simulink model "sampleModel1579_1_sub_sub"  (R2023a)
settings: Solver=VariableStepAuto  StartTime=0.0  StopTime=10.0  RelTol=1e-3
libraries: hdlsllib x7, simulink x2
settings Model: Creator=user1  LastModifiedBy=user1
settings OptimizationCC: BlockReduction=off  ConditionallyExecuteInputs=off

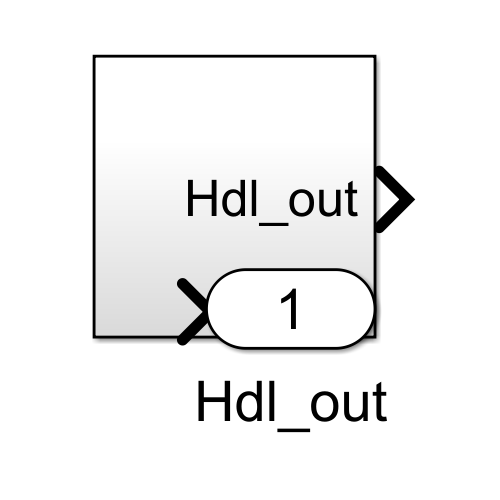
[thumbnail: Simulink's stored preview of the top-level diagram]
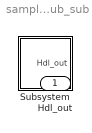
== system sampleModel1579_1_sub_sub ==
  Subsystem : Subsystem
  Hdl_out : Outport  OutDataTypeStr=uint8

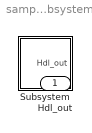
== system sampleModel1579_1_sub_sub/Subsystem ==
  Subsystem : Subsystem
  Hdl_out : Outport  OutDataTypeStr=uint8

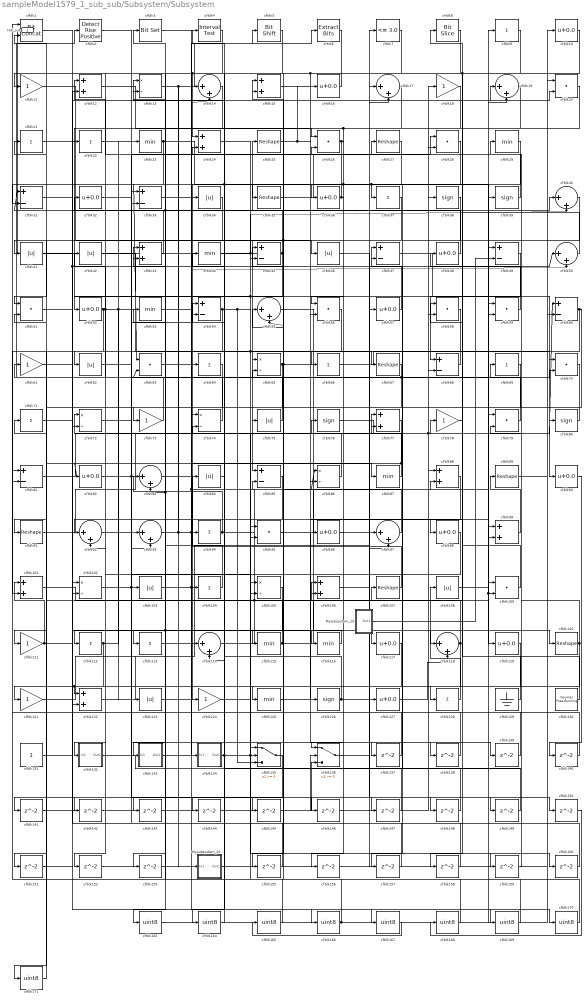
== system sampleModel1579_1_sub_sub/Subsystem/Subsystem ==
  Mysubsystem_13 : Subsystem  TreatAsAtomicUnit=on  RTWFcnName=Mysubsystem_13
      settings: RTWFcnNameOpts=User specified  RTWFileNameOpts=Use function name
  Mysubsystem_20 : Subsystem  TreatAsAtomicUnit=on  RTWFcnName=Mysubsystem_20
      settings: RTWFcnNameOpts=User specified  RTWFileNameOpts=Use function name
  cfblk1 : hdlsllib/Logic and Bit Operations/Bit Concat  numInputs=2
  cfblk{10,16,32,36,48,52,57,82,90,96,98,117,119,127} (14 alike) : Bias  Bias=0.0  SaturateOnIntegerOverflow=off
  cfblk{12,15,24,43,77,88,99,101,106,122} (10 alike) : Sum  OutDataTypeStr=uint8
  cfblk{13,65,72,74,86,102,105} (7 alike) : Product  Inputs=*/  OutDataTypeStr=uint8  RndMeth=Zero  SaturateOnIntegerOverflow=on
  cfblk{34,41..42,46,62,75,84,103,108,123} (10 alike) : Abs  OutDataTypeStr=uint8  SaturateOnIntegerOverflow=off
  cfblk{9,21..22,37,64,66,69,71,94,104,112..113,128} (13 alike) : Sum  Inputs=+  OutDataTypeStr=uint8
  cfblk{25,27,35,67,89,91,107,120} (8 alike) : Reshape
  cfblk{20,26,28,51,56,58..59,63,70,79,95,109} (12 alike) : DotProduct  OutDataTypeStr=uint8
  cfblk{11,18,61,73,78,111,121,124} (8 alike) : Gain  OutDataTypeStr=uint8
  cfblk{14,17,19,40,50,55,83,92..93,97,114,118} (12 alike) : Sum  Inputs=|++  OutDataTypeStr=uint8
  cfblk{23,29,44,53,87,115..116,125} (8 alike) : MinMax  OutDataTypeStr=uint8
  cfblk{38..39,76,80,126} (5 alike) : Signum
  cfblk129 : Ground
  cfblk130 : hdlsllib/Sources/Counter Free-Running  NumBits=16  tsamp=-1
  cfblk131 : Constant  OutDataTypeStr=uint8  SampleTime=-1
  cfblk132 : Subsystem
      settings: LibrarySourceBlock=|
      | hdlsllib/Ports &
      | Subsystems/Subsystem
  cfblk133 : Subsystem
      settings: LibrarySourceBlock=|
      | hdlsllib/Ports &
      | Subsystems/Subsystem
  cfblk134 : Subsystem
      settings: LibrarySourceBlock=|
      | hdlsllib/Ports &
      | Subsystems/Subsystem
  cfblk135 : Switch  OutDataTypeStr=uint8  SaturateOnIntegerOverflow=off  InputSameDT=off
  cfblk136 : Switch  OutDataTypeStr=uint8  SaturateOnIntegerOverflow=off  InputSameDT=off
  cfblk{137..153,155..160} (23 alike) : Delay  SampleTime=1
  cfblk{163..171} (9 alike) : DataTypeConversion  OutDataTypeStr=uint8  SaturateOnIntegerOverflow=off  RndMeth=Floor
  cfblk2 : hdlsllib/Logic and Bit Operations/Detect Rise Positive  vinit=0  OutDataTypeStr=uint8
  cfblk3 : simulink/Logic and Bit Operations/Bit Set  iBit=0
      settings: LibrarySourceBlock=|
      | hdlsllib/Logic and Bit
      | Operations/Bit Set
  cfblk{31,33,45,47,49,54,60,68,81,85} (10 alike) : Sum  Inputs=+-  OutDataTypeStr=uint8
  cfblk4 : hdlsllib/Logic and Bit Operations/Interval Test  IntervalClosedRight=on  uplimit=0.5  IntervalClosedLeft=on  lowlimit=-0.5  OutDataTypeStr=uint8
  cfblk5 : hdlsllib/Logic and Bit Operations/Bit Shift  mode=Shift Left Logical  N=0
  cfblk6 : simulink/Logic and Bit Operations/Extract Bits  bitsToExtract=Upper half  numBits=8  bitIdxRange=[0 7]  outScalingMode=Preserve fixed-point scaling
      settings: LibrarySourceBlock=|
      | hdlsllib/Logic and Bit
      | Operations/Extract Bits
  cfblk7 : hdlsllib/Logic and Bit Operations/Compare To Constant  relop=<=  const=3.0  OutDataTypeStr=uint8
  cfblk8 : hdlsllib/Logic and Bit Operations/Bit Slice  lidx=7  ridx=0
  Hdl_out : Outport  OutDataTypeStr=uint8
  wires:
  Mysubsystem_20/1(Out1) -> cfblk99/1
  Mysubsystem_13/1(Out1) -> cfblk49/2
  cfblk171/1 -> cfblk71/1
  cfblk170/1 -> cfblk55/1
  cfblk71/1 -> cfblk170/1
  cfblk169/1 -> cfblk1/2
  cfblk151/1 -> cfblk169/1
  cfblk168/1 -> cfblk1/1
  cfblk150/1 -> cfblk168/1
  cfblk167/1 -> cfblk165/1
  cfblk1/1 -> cfblk167/1
  cfblk166/1 -> cfblk109/2, cfblk79/1, cfblk135/1
  cfblk165/1 -> cfblk3/1
  cfblk164/1 -> cfblk4/1
  cfblk84/1 -> cfblk164/1
  cfblk163/1 -> cfblk10/1
  cfblk4/1 -> cfblk163/1
  cfblk160/1 -> cfblk15/2
  cfblk159/1 -> cfblk79/2
  cfblk158/1 -> cfblk102/1
  cfblk78/1 -> cfblk158/1
  cfblk157/1 -> cfblk33/1
  cfblk28/1 -> cfblk157/1
  cfblk156/1 -> cfblk19/2
  cfblk155/1 -> cfblk114/2
  cfblk153/1 -> cfblk20/1
  cfblk119/1 -> cfblk153/1
  cfblk152/1 -> cfblk97/2
  cfblk5/1 -> cfblk152/1
  cfblk149/1 -> cfblk105/1
  cfblk106/1 -> cfblk149/1
  cfblk148/1 -> cfblk47/2
  cfblk147/1 -> cfblk54/2
  cfblk2/1 -> cfblk147/1
  cfblk146/1 -> cfblk88/1
  cfblk124/1 -> cfblk146/1
  cfblk145/1 -> cfblk58/2
  cfblk56/1 -> cfblk145/1
  cfblk144/1 -> cfblk17/2
  cfblk143/1 -> cfblk136/3
  cfblk142/1 -> cfblk68/2
  cfblk85/1 -> cfblk142/1
  cfblk141/1 -> cfblk136/2
  cfblk135/1 -> cfblk141/1
  cfblk140/1 -> cfblk77/2
  cfblk90/1 -> cfblk140/1
  cfblk139/1 -> cfblk65/2
  cfblk138/1 -> cfblk81/1
  cfblk96/1 -> cfblk138/1
  cfblk137/1 -> cfblk51/2
  cfblk72/1 -> cfblk137/1
  cfblk118/1 -> cfblk21/1, cfblk135/2
  cfblk125/1 -> cfblk96/1
  cfblk95/1 -> cfblk7/1
  cfblk126/1 -> cfblk17/1, cfblk13/2
  cfblk53/1 -> cfblk67/1
  cfblk105/1 -> cfblk133/1(In1), cfblk122/2
  cfblk19/1 -> cfblk36/1, cfblk86/2
  cfblk66/1 -> cfblk70/1
  cfblk58/1 -> cfblk81/2, cfblk95/2
  cfblk16/1 -> cfblk11/1
  cfblk123/1 -> cfblk20/2
  cfblk52/1 -> cfblk95/1, cfblk123/1, cfblk92/1, cfblk101/2
  cfblk64/1 -> cfblk83/2, cfblk143/1
  cfblk133/1(Out1) -> cfblk86/1, cfblk50/2
  cfblk131/1 -> cfblk40/1, cfblk50/1
  cfblk41/1 -> cfblk12/2
  cfblk32/1 -> cfblk93/2
  cfblk136/1 -> cfblk57/1
  cfblk122/1 -> cfblk5/1
  cfblk120/1 -> cfblk29/1, cfblk171/1
  cfblk13/1 -> Mysubsystem_20/1(In1), cfblk6/1
  cfblk70/1 -> cfblk102/2
  cfblk88/1 -> cfblk104/1
  cfblk3/1 -> cfblk166/1
  cfblk83/1 -> cfblk85/2
  cfblk89/1 -> cfblk60/2
  cfblk91/1 -> cfblk39/1
  cfblk127/1 -> cfblk118/2
  cfblk50/1 -> cfblk8/1
  cfblk62/1 -> cfblk105/2
  cfblk82/1 -> cfblk60/1, cfblk28/2, cfblk115/1, cfblk70/2
  cfblk44/1 -> cfblk59/2, cfblk160/1, cfblk40/2
  cfblk51/1 -> cfblk114/1
  cfblk25/1 -> cfblk16/1, cfblk139/1
  cfblk38/1 -> cfblk72/2, cfblk55/2
  cfblk113/1 -> cfblk107/1
  cfblk59/1 -> cfblk48/1
  cfblk80/1 -> cfblk75/1
  cfblk29/1 -> cfblk45/2, cfblk156/1, cfblk37/1
  cfblk31/1 -> cfblk118/1
  cfblk129/1 -> cfblk24/2
  cfblk23/1 -> cfblk119/1, cfblk31/2
  cfblk103/1 -> cfblk134/1(In1), cfblk28/1
  cfblk77/1 -> cfblk121/1
  cfblk47/1 -> cfblk109/1
  cfblk79/1 -> cfblk15/1
  cfblk101/1 -> cfblk106/2
  cfblk121/1 -> cfblk88/2
  cfblk97/1 -> cfblk45/1
  cfblk24/1 -> cfblk120/1
  cfblk69/1 -> cfblk111/1
  cfblk34/1 -> cfblk51/1
  cfblk10/1 -> cfblk24/1, cfblk33/2, cfblk98/1
  cfblk134/1(Out1) -> cfblk76/1, cfblk159/1, cfblk74/2
  cfblk109/1 -> cfblk58/1
  cfblk115/1 -> cfblk18/1, cfblk53/1
  cfblk63/1 -> cfblk64/1
  cfblk46/1 -> cfblk127/1
  cfblk60/1 -> cfblk91/1, cfblk80/1
  cfblk12/1 -> cfblk26/1
  cfblk61/1 -> cfblk19/1
  cfblk98/1 -> cfblk132/1(In1)
  cfblk35/1 -> cfblk27/1
  cfblk18/1 -> cfblk66/1
  cfblk9/1 -> cfblk128/1
  cfblk130/1 -> cfblk106/1
  cfblk57/1 -> cfblk47/1
  cfblk6/1 -> cfblk74/1
  cfblk94/1 -> cfblk59/1, cfblk83/1
  cfblk112/1 -> cfblk122/1, cfblk151/1, cfblk23/1
  cfblk87/1 -> cfblk82/1, cfblk44/1
  cfblk37/1 -> cfblk41/1
  cfblk111/1 -> cfblk43/2, cfblk101/1
  cfblk45/1 -> cfblk13/1, cfblk31/1, cfblk52/1, Hdl_out/1
  cfblk116/1 -> cfblk113/1
  cfblk8/1 -> cfblk65/1, cfblk56/2
  cfblk132/1(Out1) -> cfblk69/1
  cfblk39/1 -> cfblk12/1
  cfblk117/1 -> cfblk125/1
  cfblk42/1 -> cfblk97/1
  cfblk108/1 -> cfblk49/1
  cfblk67/1 -> cfblk63/2, cfblk92/2
  cfblk74/1 -> cfblk43/1
  cfblk76/1 -> cfblk78/1
  cfblk86/1 -> cfblk72/1
  cfblk92/1 -> cfblk54/1
  cfblk22/1 -> cfblk93/1
  cfblk128/1 -> cfblk108/1
  cfblk75/1 -> cfblk42/1
  cfblk33/1 -> cfblk87/1
  cfblk14/1 -> cfblk112/1
  cfblk65/1 -> cfblk99/2, cfblk155/1, cfblk94/1
  cfblk68/1 -> cfblk62/1
  cfblk54/1 -> cfblk135/3, cfblk148/1, cfblk73/1
  cfblk114/1 -> cfblk38/1, cfblk9/1
  cfblk107/1 -> cfblk84/1
  cfblk36/1 -> cfblk34/1, cfblk116/1
  cfblk17/1 -> cfblk136/1
  cfblk49/1 -> cfblk68/1
  cfblk99/1 -> cfblk89/1
  cfblk93/1 -> cfblk14/2, cfblk150/1, cfblk14/1
  cfblk102/1 -> cfblk103/1, cfblk26/2
  cfblk20/1 -> cfblk22/1
  cfblk40/1 -> cfblk85/1
  cfblk7/1 -> cfblk35/1
  cfblk104/1 -> cfblk61/1
  cfblk26/1 -> cfblk63/1, cfblk144/1, cfblk56/1
  cfblk48/1 -> cfblk25/1
  cfblk15/1 -> cfblk126/1
  cfblk81/1 -> cfblk77/1
  cfblk43/1 -> cfblk32/1
  cfblk27/1 -> cfblk124/1
  cfblk21/1 -> cfblk90/1
  cfblk73/1 -> cfblk2/1
  cfblk55/1 -> cfblk117/1
  cfblk11/1 -> cfblk46/1

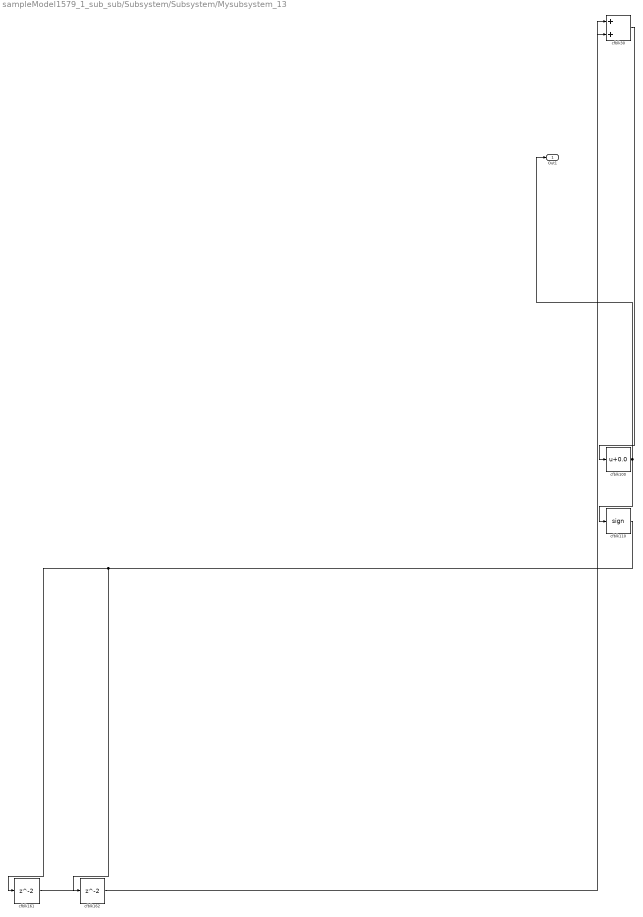
== system sampleModel1579_1_sub_sub/Subsystem/Subsystem/Mysubsystem_13 ==
  cfblk100 : Bias  Bias=0.0  SaturateOnIntegerOverflow=off
  cfblk110 : Signum
  cfblk161 : Delay  SampleTime=1
  cfblk162 : Delay  SampleTime=1
  cfblk30 : Sum
  Out1 : Outport
  wires:
  cfblk161/1 -> cfblk30/1
  cfblk30/1 -> cfblk100/1
  cfblk110/1 -> cfblk161/1, cfblk162/1
  cfblk162/1 -> cfblk30/2
  cfblk100/1 -> Out1/1, cfblk110/1

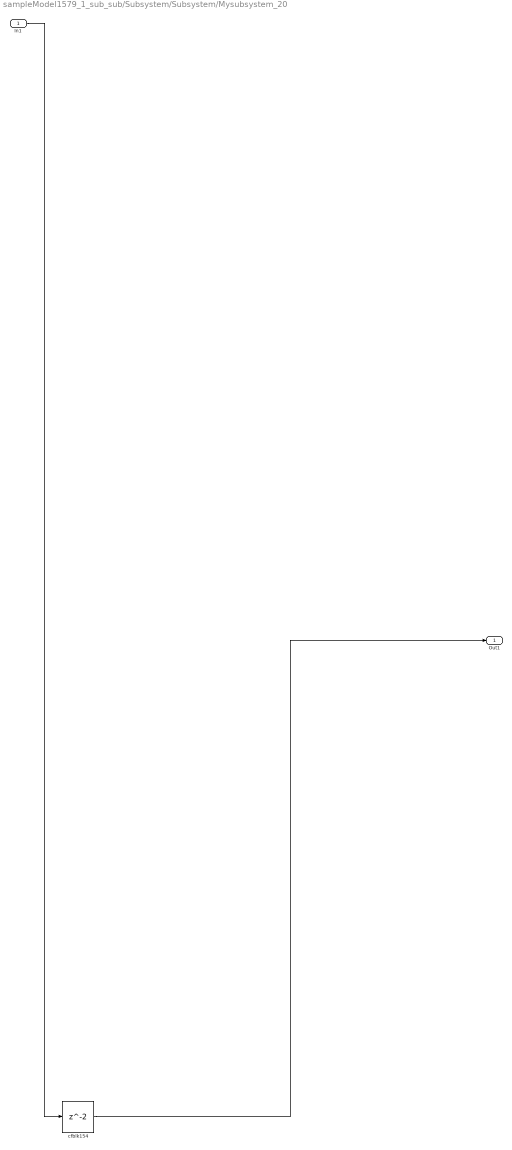
== system sampleModel1579_1_sub_sub/Subsystem/Subsystem/Mysubsystem_20 ==
  In1 : Inport
  cfblk154 : Delay  SampleTime=1
  Out1 : Outport
  wires:
  In1/1 -> cfblk154/1
  cfblk154/1 -> Out1/1

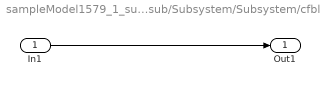
== system sampleModel1579_1_sub_sub/Subsystem/Subsystem/cfblk132 ==
  In1 : Inport
  Out1 : Outport
  wires:
  In1/1 -> Out1/1

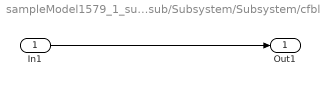
== system sampleModel1579_1_sub_sub/Subsystem/Subsystem/cfblk133 ==
  In1 : Inport
  Out1 : Outport
  wires:
  In1/1 -> Out1/1

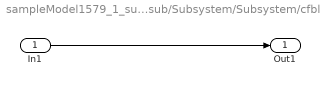
== system sampleModel1579_1_sub_sub/Subsystem/Subsystem/cfblk134 ==
  In1 : Inport
  Out1 : Outport
  wires:
  In1/1 -> Out1/1
